simulink model "TresIngestasPS"  (R2024b)
settings: Solver=VariableStepAuto  StartTime=0.0  StopTime=120000  RelTol=1e-3
undefined symbols (not defined in the file): n, p1, p2, p3, Vi
libraries: slpidlib x1
settings Model: Creator=HP  LastModifiedBy=HP

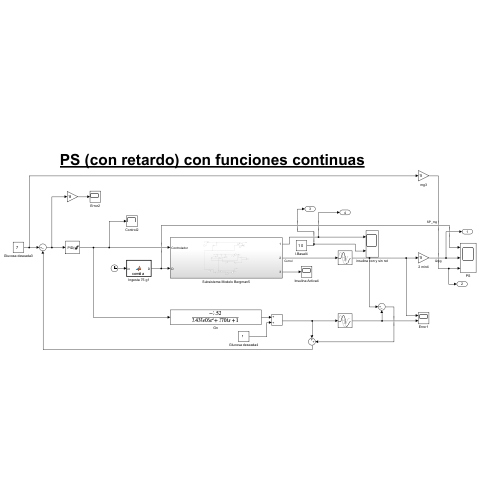
[thumbnail: Simulink's stored preview of the top-level diagram]
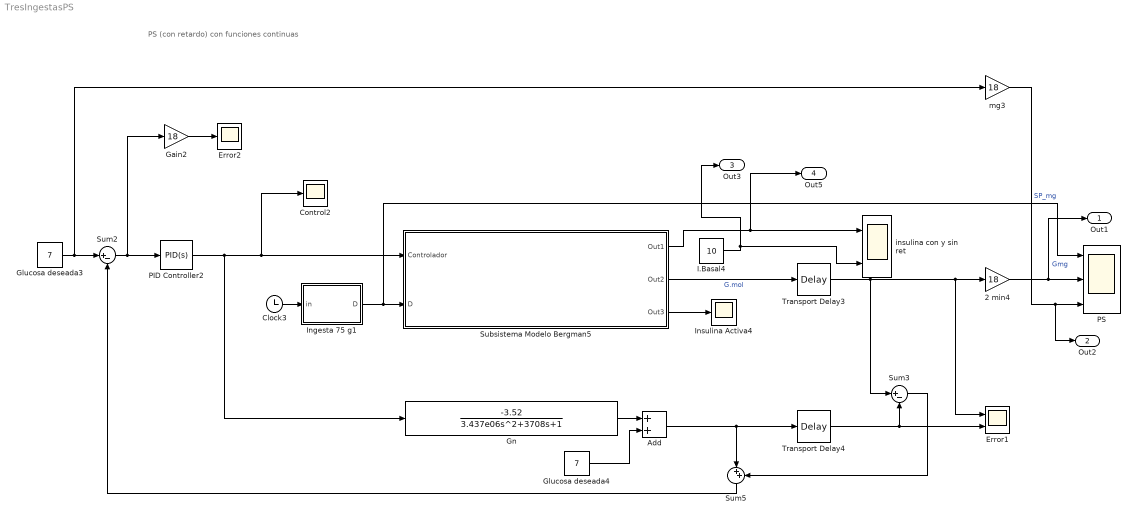
== system TresIngestasPS ==
  note: PS (con retardo) con funciones continuas
  2 min4 : Gain  Gain=18
  Add : Sum
  Clock3 : Clock
  Control2 : Scope
  Error1 : Scope  NumInputPorts=2
  Error2 : Scope
  Gain2 : Gain  Gain=18
  Glucosa deseada3 : Constant  Value=7
  Glucosa deseada4 : Constant  Value=7
  Gn : TransferFcn  Numerator=[-3.52]  Denominator=[3.437e06 3708 1]
  I.Basal4 : Constant  Value=10
  Ingesta 75 g1 : MATLAB Function  TreatAsAtomicUnit=on
  Insulina Activa4 : Scope
  PID Controller2 : slpidlib/PID Controller  Controller=PID  Form=Parallel  TimeDomain=Continuous-time  UseExternalTs=off  SampleTime=-1  IntegratorMethod=Forward Euler  FilterMethod=Forward Euler  ControllerParametersSource=internal  P=-0.3195*1.5  I=-0.3195/2998.95  UseKiTs=off  D=0  UseExternalDerivativeSource=off  N=10  UseFilter=on  TunerSelectOption=Transfer Function Based (PID Tuner App)  InitialConditionSource=internal  InitialConditionForIntegrator=0  InitialConditionForFilter=0  DifferentiatorICPrevScaledInput=0  ExternalReset=none  TrackingMode=off  Kt=1  LimitOutput=on  SatLimitsSource=internal  UpperSaturationLimit=5  LowerSaturationLimit=0  LinearizeAsGain=on  AntiWindupMode=none  Kb=1  LimitIntegrator=off  UpperIntegratorSaturationLimit=inf  LowerIntegratorSaturationLimit=-inf  POutMin=[]  POutMax=[]  IOutMin=[]  IOutMax=[]  DOutMin=[]  DOutMax=[]  NOutMin=[]  NOutMax=[]  SumOutMin=[]  SumOutMax=[]  SaturationOutMin=[]  SaturationOutMax=[]  PParamMin=[]  PParamMax=[]  IParamMin=[]  IParamMax=[]  DParamMin=[]  DParamMax=[]  NParamMin=[]  NParamMax=[]  KbParamMin=[]  KbParamMax=[]  KtParamMin=[]  KtParamMax=[]  KbOutMin=[]  KbOutMax=[]  KtOutMin=[]  KtOutMax=[]  IntegratorOutMin=[]  IntegratorOutMax=[]  FilterOutMin=[]  FilterOutMax=[]  SumI1OutMin=[]  SumI1OutMax=[]  SumI2OutMin=[]  SumI2OutMax=[]  SumI3OutMin=[]  SumI3OutMax=[]  SumI4OutMin=[]  SumI4OutMax=[]  SumDOutMin=[]  SumDOutMax=[]  DifferentiatorOutMin=[]  DifferentiatorOutMax=[]  FilterDiffOutCoefMin=[]  FilterDiffOutCoefMax=[]  ReciprocalOutMin=[]  ReciprocalOutMax=[]  SumDenOutMin=[]  SumDenOutMax=[]  SumNumOutMin=[]  SumNumOutMax=[]  DivideOutMin=[]  DivideOutMax=[]  UdiffTsProdOutMin=[]  UdiffTsProdOutMax=[]  NTsProdOutMin=[]  NTsProdOutMax=[]  UintegralTsProdOutMin=[]  UintegralTsProdOutMax=[]  UngainTsProdOutMin=[]  UngainTsProdOutMax=[]  ClampingZeroOutDataTypeStr=Inherit: Inherit via back propagation  ClampingZeroOutMin=[]  ClampingZeroOutMax=[]  FilterDenConstantOutDataTypeStr=Inherit: Inherit via back propagation  FilterDenConstantOutMin=[]  FilterDenConstantOutMax=[]  PCopyOutDataTypeStr=Inherit: Inherit via back propagation  PCopyOutMin=[]  PCopyOutMax=[]  NCopyOutDataTypeStr=Inherit: Inherit via back propagation  NCopyOutMin=[]  NCopyOutMax=[]  IntegratorContinuousStateAttributes=''  IntegratorStateMustResolveToSignalObject=off  IntegratorRTWStateStorageClass=Auto  FilterContinuousStateAttributes=''  FilterStateMustResolveToSignalObject=off  FilterRTWStateStorageClass=Auto  ParallelPVariant=InternalParameters  IdealPVariant=Disabled  IVariant=InternalParameters  DVariant=InternalParameters  IntegratorVariant=Continuous  SatVariant=Enabled  AWVariant=Passthrough  PCopyVariant=Disabled  TRVariant=Disabled  FdbkBlocksVariant=Forward  IdealPFdbkVariant=Disabled  SatFdbkVariant=Disabled  DerivativeFilterVariant=ContFilter  NVariant=InternalParameters  NCopyVariant=Disabled  FilterICVariant=InternalICsFilter  IntegratorICVariant=InternalICs  ExternalResetVariant=Disabled  TRSumVariant=Passthrough  SumFdbkVariant=Disabled  SumVariant=Sum_PID  TsampFilterVariant=InternalTs  TsampNgainVariant=Passthrough  TsampIntegralVariant=Disabled_SignalSpec  ExternalSaturationOutDataTypeStr=Inherit: Same as second input  DerivativeSourceVariant=ErrorSignal  PreIntVariant=InternalPreInt
  PS : Scope  NumInputPorts=3
  Subsistema Modelo Bergman5 : Subsystem
  Sum2 : Sum  Inputs=|+-
  Sum3 : Sum  Inputs=|+-
  Sum5 : Sum  Inputs=|++
  Transport Delay3 : TransportDelay  DelayTime=900  InitialOutput=7
  Transport Delay4 : TransportDelay  DelayTime=900  InitialOutput=7
  insulina con y sin ret : Scope  NumInputPorts=2
  mg3 : Gain  Gain=18
  Out1 : Outport
  Out2 : Outport  Port=2
  Out3 : Outport  Port=3
  Out5 : Outport  Port=4
  wires:
  Sum2/1 -> Gain2/1, PID Controller2/1
  Transport Delay3/1 -> Sum3/1, Error1/1, 2 min4/1
  mg3/1 -> Out2/1, PS/3  "SP_mg"
  Glucosa deseada3/1 -> mg3/1, Sum2/1
  Clock3/1 -> Ingesta 75 g1/1(in)
  Subsistema Modelo Bergman5/3(Out3) -> Insulina Activa4/1
  Subsistema Modelo Bergman5/2(Out2) -> Transport Delay3/1  "G.mol"
  Subsistema Modelo Bergman5/1(Out1) -> Out5/1, insulina con y sin ret/1
  Ingesta 75 g1/1(D) -> PS/1, Subsistema Modelo Bergman5/2(D)
  PID Controller2/1 -> Gn/1, Control2/1, Subsistema Modelo Bergman5/1(Controlador)
  Gn/1 -> Add/1
  I.Basal4/1 -> Out3/1, insulina con y sin ret/2
  Sum3/1 -> Sum5/2
  Glucosa deseada4/1 -> Add/2
  Gain2/1 -> Error2/1
  Add/1 -> Transport Delay4/1, Sum5/1
  Transport Delay4/1 -> Sum3/2, Error1/2
  2 min4/1 -> Out1/1, PS/2  "Gmg"
  Sum5/1 -> Sum2/2

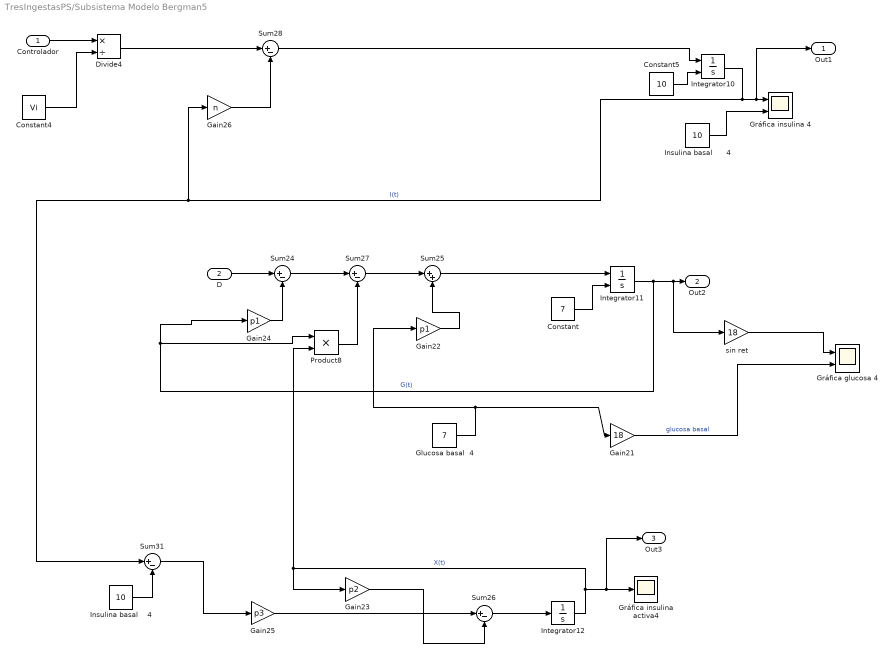
== system TresIngestasPS/Subsistema Modelo Bergman5 ==
  Controlador : Inport
  D : Inport  Port=2
  Constant : Constant  Value=7
  Constant4 : Constant  Value=Vi
  Constant5 : Constant  Value=10
  Divide4 : Product  Inputs=*/
  Gain21 : Gain  Gain=18
  Gain22 : Gain  Gain=p1
  Gain23 : Gain  Gain=p2
  Gain24 : Gain  Gain=p1
  Gain25 : Gain  Gain=p3
  Gain26 : Gain  Gain=n
  Glucosa basal  4 : Constant  Value=7
  Gráfica glucosa 4 : Scope  NumInputPorts=2
  Gráfica insulina 4 : Scope  NumInputPorts=2
  Gráfica insulina activa4 : Scope
  Insulina basal      4 : Constant  Value=10
  Insulina basal    4 : Constant  Value=10
  Integrator10 : Integrator  InitialConditionSource=external
  Integrator11 : Integrator  InitialConditionSource=external  InitialCondition=7
  Integrator12 : Integrator
  Product8 : Product
  Sum{24,26..28,31} (5 alike) : Sum  Inputs=|+-
  Sum25 : Sum  Inputs=|++
  sin ret : Gain  Gain=18
  Out1 : Outport
  Out2 : Outport  Port=2
  Out3 : Outport  Port=3
  wires:
  Gain26/1 -> Sum28/2
  Glucosa basal  4/1 -> Gain22/1, Gain21/1
  D/1 -> Sum24/1
  Gain21/1 -> Gráfica glucosa 4/2  "glucosa basal"
  Integrator11/1 -> sin ret/1, Out2/1, Gain24/1, Product8/1  "G(t)"
  Integrator12/1 -> Product8/2, Gain23/1, Out3/1, Gráfica insulina activa4/1  "X(t)"
  Gain25/1 -> Sum26/1
  Integrator10/1 -> Out1/1, Gráfica insulina 4/1, Sum31/1, Gain26/1  "I(t)"
  Constant5/1 -> Integrator10/2
  Sum31/1 -> Gain25/1
  Sum26/1 -> Integrator12/1
  Gain23/1 -> Sum26/2
  Sum28/1 -> Integrator10/1
  Sum24/1 -> Sum27/1
  Sum25/1 -> Integrator11/1
  Gain24/1 -> Sum24/2
  Insulina basal      4/1 -> Gráfica insulina 4/2
  Sum27/1 -> Sum25/1
  Insulina basal    4/1 -> Sum31/2
  Divide4/1 -> Sum28/1
  Gain22/1 -> Sum25/2
  Product8/1 -> Sum27/2
  Constant4/1 -> Divide4/2
  Constant/1 -> Integrator11/2
  Controlador/1 -> Divide4/1
  sin ret/1 -> Gráfica glucosa 4/1

== matlab function TresIngestasPS/Ingesta 75 g1 ==
  data: in input; D output
function D = comida(in)
% Variables de entrada en la función
t = in(1); % Tiempo en segundos

% Parámetros del modelo
Ag = 0.8; % adimensional
Tmaxi = 55*60; % s
Vg = 13.79; % L
Tmaxg = 40*60; % s

% Tiempo de inicio para cada comida
t1 = 6 * 60 * 60; % Desayuno
t2 = 13.5 * 60 * 60; % Almuerzo
t3 = 23 * 60 * 60; % Cena

% Cantidad de glucosa ingerida (en mmol, ajustado según el factor de conversión)
Dg1 = 10 * (1000/180); % Desayuno
Dg2 = 35 * (1000/180); % Almuerzo
Dg3 = 20 * (1000/180); % Cena

% Ecuación desayuno
if t >= t1 && t < t2
    D = (Dg1 * Ag * (t - t1) * exp(-(t - t1) / Tmaxi)) / (Vg * Tmaxg^2);
% Ecuación almuerzo
elseif t >= t2 && t < t3
    D = (Dg1 * Ag * (t - t1) * exp(-(t - t1) / Tmaxi)) / (Vg * Tmaxg^2) + ...
        (Dg2 * Ag * (t - t2) * exp(-(t - t2) / Tmaxi)) / (Vg * Tmaxg^2);
% Ecuación cena
elseif t >= t3
    D = (Dg1 * Ag * (t - t1) * exp(-(t - t1) / Tmaxi)) / (Vg * Tmaxg^2) + ...
        (Dg2 * Ag * (t - t2) * exp(-(t - t2) / Tmaxi)) / (Vg * Tmaxg^2) + ...
        (Dg3 * Ag * (t - t3) * exp(-(t - t3) / Tmaxi)) / (Vg * Tmaxg^2);
else
    D = 0;
end
end
